simulink model "AnalogSwitchTest"  (R2016a)
settings: Solver=VariableStepAuto  StartTime=0.0  StopTime=1  RelTol=1e-3
libraries: SimscapeMacros x4, fl_lib x3, ProjectBlocks x1, nesl_utility x1
settings Model: Creator=Peter  LastModifiedBy=Peter

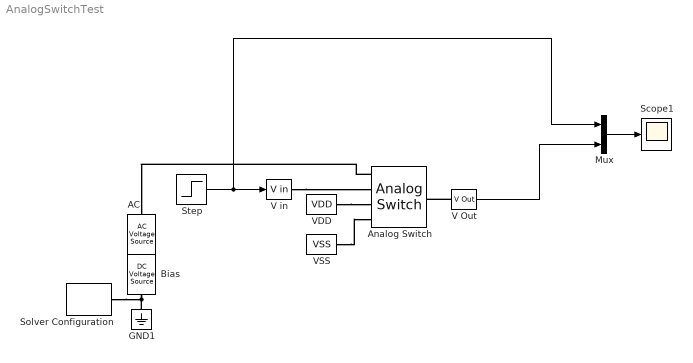
== system AnalogSwitchTest ==
  AC : fl_lib/Electrical/Electrical Sources/AC Voltage Source  amp=5 V  shift=0 deg  frequency=10 Hz  omega=0 rad/s
  Analog Switch : ProjectBlocks/Analog Switch
  Bias : fl_lib/Electrical/Electrical Sources/DC Voltage Source  v0=0 V
  GND1 : fl_lib/Electrical/Electrical Elements/Electrical Reference
  Mux : Mux  Inputs=2
  Scope1 : Scope
  Solver Configuration : nesl_utility/Solver Configuration  PhysicalDomain=network_engine_domain  SubClassName=solver  LeftPortType=input  RightPortType=generic  Accelerate=off  Tones=[]  Harmonics=[]  SimulateNoise=off  Profile=off  UseLocalSampling=off  EnableSwitchedLinearOptims=on  FrequencyDomain=off  UseCCode=off  RelTol=0.001  AbsTol=1e-06  MinStep=1e-09  ToWorkspace=off  RevertToSquareIcSolve=off  NumHomotopyIterations=100  PhasorMode=off  PhasorModeNumHarmonics=1  OverrideAbsTol=off  DoDC=off  ResidualTolerance=1e-09  UseLocalSolver=off  LocalSolverChoice=NE_BACKWARD_EULER_ADVANCER  LocalSolverSampleTime=0.001  DoFixedCost=off  MaxNonlinIter=3  MaxModeIter=2  LinearAlgebra=Sparse  DelaysMemoryBudget=1024  AutomaticFiltering=on  FilteringTimeConstant=0.001
  Step : Step  Time=.5  Before=-10  After=10  SampleTime=0
  V Out : SimscapeMacros/V Out
  V in : SimscapeMacros/V in
  VDD : SimscapeMacros/VDD
  VSS : SimscapeMacros/VSS
  wires:
  Step/1 -> V in/1, Mux/1
  V Out/1 -> Mux/2
  Mux/1 -> Scope1/1
  connections:
  GND1/LConn1 -- Bias/RConn1 -- Solver Configuration/RConn1
  AC/RConn1 -- Bias/LConn1
  Analog Switch/LConn1 -- AC/LConn1
  V Out/LConn1 -- Analog Switch/RConn1
  V in/RConn1 -- Analog Switch/LConn2
  VDD/RConn1 -- Analog Switch/LConn3
  VSS/RConn1 -- Analog Switch/LConn4
